simulink model "Test_BlockIO"  (R2020a)
settings: configuration reference "testConfig" (kept outside this file)
undefined symbols (not defined in the file or in its folder): DiscIntNeverNeededParam
settings Model: DataDictionary=TestConfig.sldd  Creator=toma  LastModifiedBy=toma
settings ConfigSetRef: SourceName=testConfig

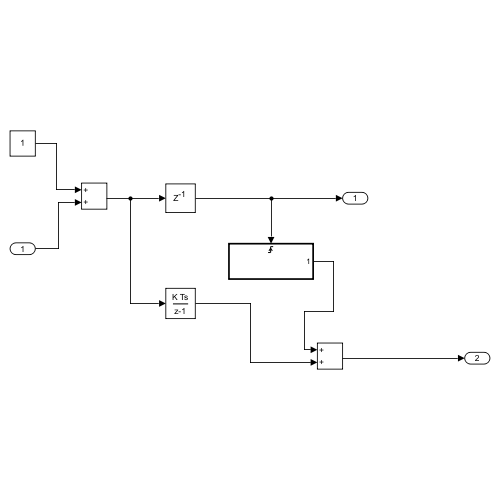
[thumbnail: Simulink's stored preview of the top-level diagram]
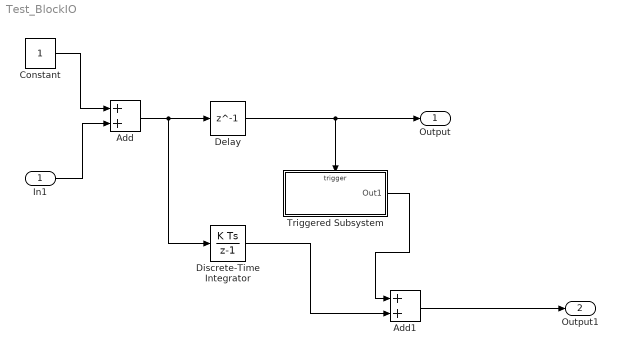
== system Test_BlockIO ==
  In1 : Inport
  Add : Sum
  Add1 : Sum
  Constant : Constant
  Delay : Delay  DelayLength=1  InitialCondition=0
  Discrete-Time Integrator : DiscreteIntegrator  InitialCondition=5  SampleTime=-1  ICPrevOutput=DiscIntNeverNeededParam  ICPrevScaledInput=DiscIntNeverNeededParam
  Triggered Subsystem : Subsystem  TreatAsAtomicUnit=on
  Output : Outport
  Output1 : Outport  Port=2
  wires:
  In1/1 -> Add/2
  Delay/1 -> Triggered Subsystem/Trigger, Output/1
  Add/1 -> Discrete-Time Integrator/1, Delay/1
  Constant/1 -> Add/1
  Discrete-Time Integrator/1 -> Add1/2
  Add1/1 -> Output1/1
  Triggered Subsystem/1(Out1) -> Add1/1

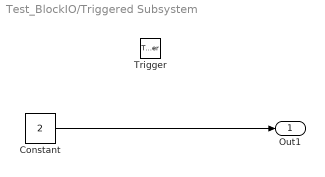
== system Test_BlockIO/Triggered Subsystem ==
  Trigger : TriggerPort  VariantControl=(inherit)  InitialTriggerSignalState=negative
  Constant : Constant  Value=2
  Out1 : Outport  InitialOutput=1
  wires:
  Constant/1 -> Out1/1
